simulink model "ASK"  (R2019a)
settings: Solver=VariableStepAuto  StartTime=0.0  StopTime=10.0  MaxStep=0.001  RelTol=1e-3
libraries: commchan3 x1, commrandsrc3 x1
settings Model: Creator=MOSA  LastModifiedBy=MOSA
settings DebuggingCC: SFMachineParentedDataDiag=error

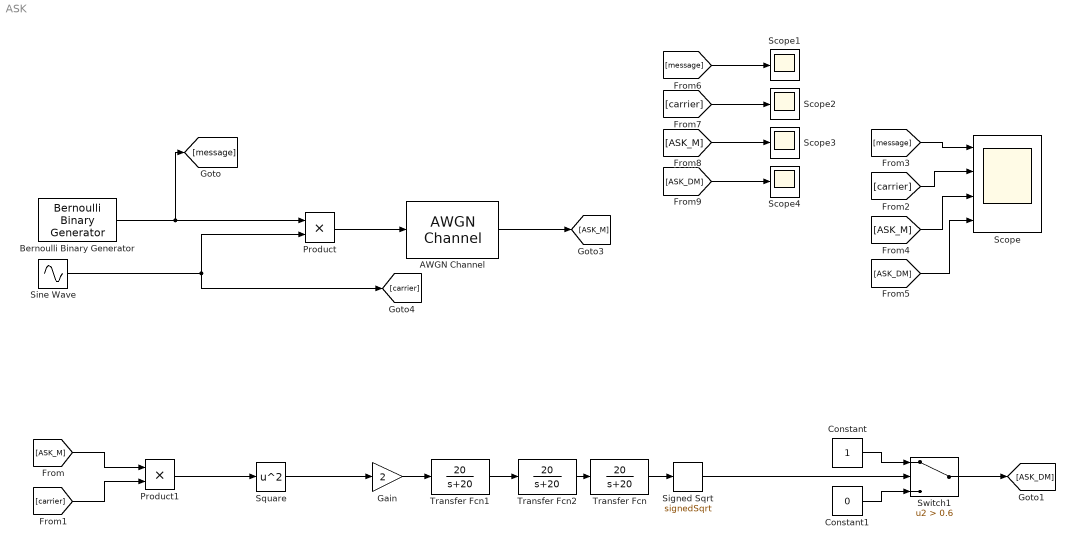
== system ASK ==
  AWGN Channel : commchan3/AWGN Channel  InputProcessing=Columns as channels (frame based)  seed=67  noiseMode="Signal to noise ratio  (SNR)"  EbNodB=10  EsNodB=10  SNRdB=10  bitsPerSym=1  Ps=1  Tsym=1  variance=1
  Bernoulli Binary Generator : commrandsrc3/Bernoulli Binary Generator  ProbabilityOfZero=0.5  SeedSource=Parameter  Seed=67  SampleTime=0.4  SamplesPerFrame=1  OutputDataType=double  SimulateUsing=Interpreted execution
  Constant : Constant
  Constant1 : Constant  Value=0
  Gain : Gain  Gain=2
  Product : Product
  Product1 : Product
  Scope : Scope  NumInputPorts=4
  Scope{1..4} (4 alike) : Scope
  Signed Sqrt : Sqrt  Operator=signedSqrt  SaturateOnIntegerOverflow=on
  Sine Wave : Sin  Frequency=2*pi*5  SampleTime=0
  Square : Math  Operator=square  SaturateOnIntegerOverflow=on
  Switch1 : Switch  Criteria=u2 > Threshold  Threshold=0.6
  Transfer Fcn : TransferFcn  Numerator=[20]  Denominator=[1 20]
  Transfer Fcn1 : TransferFcn  Numerator=[20]  Denominator=[1 20]
  Transfer Fcn2 : TransferFcn  Numerator=[20]  Denominator=[1 20]
  wires:
  Bernoulli Binary Generator/1 -> [message], Product/1
  [message] -> Scope/1
  [carrier] -> Scope/2
  Sine Wave/1 -> [carrier], Product/2
  Product1/1 -> Square/1
  [ASK_M] -> Product1/1
  Product/1 -> AWGN Channel/1
  [carrier] -> Product1/2
  [ASK_M] -> Scope/3
  [ASK_DM] -> Scope/4
  Gain/1 -> Transfer Fcn1/1
  Square/1 -> Gain/1
  Transfer Fcn2/1 -> Transfer Fcn/1
  Transfer Fcn1/1 -> Transfer Fcn2/1
  Transfer Fcn/1 -> Signed Sqrt/1
  Constant1/1 -> Switch1/3
  Signed Sqrt/1 -> Switch1/2
  Constant/1 -> Switch1/1
  Switch1/1 -> [ASK_DM]
  AWGN Channel/1 -> [ASK_M]
  [message] -> Scope1/1
  [ASK_DM] -> Scope4/1
  [ASK_M] -> Scope3/1
  [carrier] -> Scope2/1
